simulink library "NiCiDuty"  (Simulink 7.8)
settings: Solver=ode45  StartTime=0.0  StopTime=10.0  RelTol=1e-3
settings Model: Creator=Administrator  LastModifiedBy=KLJS168

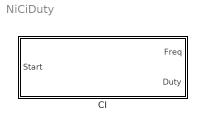
== system NiCiDuty ==
  CI : Subsystem  mask(CI){devid=0, chanid=0}
      mask prompts: chanid "Channel ID"
      mask help:
      | Dev ID
      |     You can find the ID by nilsdev commond after you install DAQmx.
      | Channel ID
      |     Specify the channel you want to use .
      mask init:
      | displayblock=sprintf('\nCI Duty\nDev ID: %d Chan ID: %d\n',devid,chanid);
      mask Display: disp(displayblock);

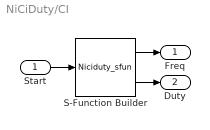
== system NiCiDuty/CI ==
  Start : Inport
  S-Function Builder : S-Function  InitFcn=try, set_param(gcb,'FunctionName','Niciduty_sfun'), end  FunctionName=Niciduty_sfun  Parameters=devid,chanid  WizardData=DataTag0  EnableBusSupport=off  mask(S-Function Builder){}
      mask help: Simulink:masks:SFunctionBuilder_MD
      mask init:
      | val = [[.9  0.75 0.75 1 1 .9 .9 1]',[1 1 0.75 0.75 .9 .9 1 .9]'];try , sys = get_param(gcb,'SfunBuilderFcnName');if isempty(sys), sys = get_param(gcb,'FunctionName'); end,catch, sys = get_param(gcb,'FunctionName'); end
      settings: CopyFcn=set_param(gcbh,'LinkStatus','none')  PreSaveFcn=try, set_param(gcb,'FunctionName','Niciduty_sfun'), end  OpenFcn=sfunctionwizard(gcbh)
      mask Display: plot(val(:,1),val(:,2)),disp(sys), port_label('input',1,'u0'), port_label('output',1,'y0'), port_label('output',2,'y1')
  Freq : Outport
  Duty : Outport  Port=2
  wires:
  S-Function Builder/2 -> Duty/1
  Start/1 -> S-Function Builder/1
  S-Function Builder/1 -> Freq/1
